simulink model "Prvi2012B"  (R2012b)
settings: Solver=ode45  SolverMode=SingleTasking  StartTime=0.0  StopTime=20  RelTol=1e-3
settings Model: CovMetricSettings=dwe  CovHtmlReporting=off  covSaveCumulativeToWorkspaceVar=off  CovSaveSingleToWorkspaceVar=off  CovExternalEMLEnable=on  Creator=Emina  LastModifiedBy=Aldin
settings DataIOCC: LimitDataPoints=off  SaveFormat=StructureWithTime  ReturnWorkspaceOutputs=on
settings OptimizationCC: ExpressionDepthLimit=128
settings DebuggingCC: UnderspecifiedInitializationDetection=Simplified  MergeDetectMultiDrivingBlocksExec=error  SolverPrmCheckMsg=none  FrameProcessingCompatibilityMsg=error  StateNameClashWarn=none  SFUnexpectedBacktrackingDiag=error  SFNoUnconditionalDefaultTransitionDiag=error
settings HardwareCC: ProdBitPerPointer=64  ProdLargestAtomicFloat=Float  ProdIntDivRoundTo=Zero  ProdEndianess=LittleEndian  ProdHWDeviceType=Specified
settings ModelReferenceCC: PropagateSignalLabelsOutOfModel=on
settings SFSimCC: SimUseLocalCustomCode=on
settings RTWCC: RTWUseLocalCustomCode=on
settings CodeAppCC: CustomSymbolStrType=$N$R$M_T
settings GRTTargetCC: CodeReplacementLibrary=C99 (ISO)

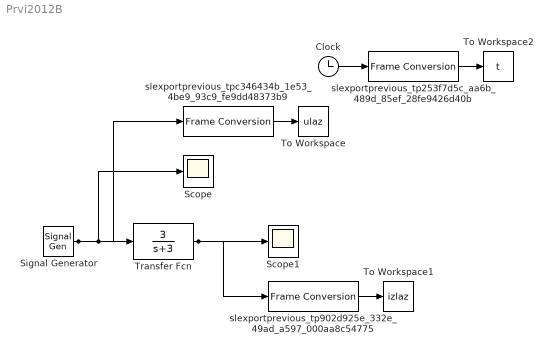
== system Prvi2012B ==
  Clock : Clock
  Scope : Scope
      settings: TimeRange=auto  MaxDataPoints=5000  SaveToWorkspace=off  SaveName=ScopeData  YMin=-1.25  YMax=1.25  SampleTime=-1
  Scope1 : Scope
      settings: TimeRange=auto  MaxDataPoints=5000  SaveToWorkspace=off  YMin=-1.2464  YMax=1.24419  SampleTime=-1
  Signal Generator : SignalGenerator  WaveForm=square  Frequency=0.25
  To Workspace : ToWorkspace  VariableName=ulaz  SampleTime=-1
  To Workspace1 : ToWorkspace  VariableName=izlaz  SampleTime=-1
  To Workspace2 : ToWorkspace  VariableName=t  SampleTime=-1
  Transfer Fcn : TransferFcn  Numerator=[3]  Denominator=[1 3]
  slexportprevious_tp253f7d5c_aa6b_489d_85ef_28fe9426d40b : FrameConversion  OutFrame=Sample-based
  slexportprevious_tp902d925e_332e_49ad_a597_000aa8c54775 : FrameConversion  OutFrame=Sample-based
  slexportprevious_tpc346434b_1e53_4be9_93c9_fe9dd48373b9 : FrameConversion  OutFrame=Sample-based
  wires:
  Signal Generator/1 -> Transfer Fcn/1, Scope/1, slexportprevious_tpc346434b_1e53_4be9_93c9_fe9dd48373b9/1
  Transfer Fcn/1 -> Scope1/1, slexportprevious_tp902d925e_332e_49ad_a597_000aa8c54775/1
  slexportprevious_tpc346434b_1e53_4be9_93c9_fe9dd48373b9/1 -> To Workspace/1
  slexportprevious_tp902d925e_332e_49ad_a597_000aa8c54775/1 -> To Workspace1/1
  Clock/1 -> slexportprevious_tp253f7d5c_aa6b_489d_85ef_28fe9426d40b/1
  slexportprevious_tp253f7d5c_aa6b_489d_85ef_28fe9426d40b/1 -> To Workspace2/1
